simulink model "control_algorithm"  (R2021a)
settings: Solver=FixedStepDiscrete  StartTime=0.0  StopTime=Inf  FixedStep=5e-05  MaxStep=1e-6  RelTol=1e-9  EnableMultiTasking=on
values from neighbouring files (symbols this model uses):
  HW_TS = PWM_PRD    (= 5e-05)    [parameters.m]
  PWM_TIM_BASE_PRD = PWM_CPU_CLK/PWM_FS    (= 5000)    [parameters.m]
  VSI_AMP = 6    [parameters.m]
  VSI_FREQ = 50    [parameters.m]
settings Model: ExtModeTrigDuration=8  Creator=61301765  LastModifiedBy=61301765
settings SolverCC: ZeroCrossAlgorithm=Adaptive
settings DataIOCC: SaveOutput=off  SaveTime=off
settings OptimizationCC: DefaultUnderspecifiedDataType=single  EnhancedBackFolding=on  PassReuseOutputArgsAs=Individual arguments  MaxStackSize=1024  OptimizeBlockOrder=speed  DifferentSizesBufferReuse=on  OptimizationCustomize=off  DenormalBehavior=FlushToZero  EfficientTunableParamExpr=on
settings DebuggingCC: ParameterTunabilityLossMsg=error
settings HardwareCC: ProdBitPerChar=16  ProdBitPerInt=16  ProdBitPerPointer=32  ProdBitPerSizeT=32  ProdBitPerPtrDiffT=32  ProdLargestAtomicInteger=Integer  ProdLargestAtomicFloat=None  ProdWordSize=16  ProdLongLongMode=on  ProdHWDeviceType=Texas Instruments->C2000
settings SFSimCC: MATLABDynamicMemAlloc=off
settings RTWCC: SystemTargetFile=ert.tlc  HardwareBoard=TI Piccolo F280049C LaunchPad  TemplateMakefile=ert_default_tmf  Toolchain=Microsoft Visual C++ 2019 v16.0 | nmake (64-bit Windows)  PortableWordSizes=on
settings CodeAppCC: ForceParamTrailComments=on  IgnoreCustomStorageClasses=off  OperatorAnnotations=on  SimulinkDataObjDesc=on  SFDataObjDesc=on  InsertBlockDesc=on
settings ERTTargetCC: CodeReplacementLibrary=TI C28x  ExtModeTransport=3  ExtModeStaticAllocSize=5000
settings SimscapeCC: SimscapeLogType=all  SimscapeLogToSDI=on  SimscapeLogLimitData=off

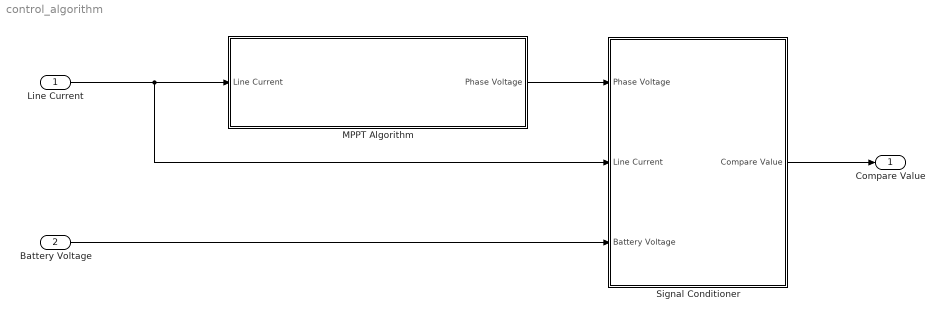
== system control_algorithm ==
  Line Current : Inport  OutDataTypeStr=double  PortDimensions=3  SampleTime=[5.0000000000000002e-05,0]
  Battery Voltage : Inport  Port=2  OutDataTypeStr=double  PortDimensions=1  SampleTime=[5.0000000000000002e-05,0]
  MPPT Algorithm : Subsystem
  Signal Conditioner : Subsystem
  Compare Value : Outport  OutDataTypeStr=uint32  PortDimensions=3  SampleTime=[5.0000000000000002e-05,0]
  wires:
  MPPT Algorithm/1(Phase Voltage) -> Signal Conditioner/1(Phase Voltage)
  Line Current/1 -> Signal Conditioner/2(Line Current), MPPT Algorithm/1(Line Current)
  Battery Voltage/1 -> Signal Conditioner/3(Battery Voltage)
  Signal Conditioner/1(Compare Value) -> Compare Value/1

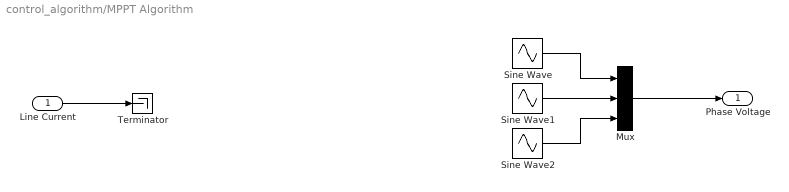
== system control_algorithm/MPPT Algorithm ==
  Line Current : Inport
  Mux : Mux  Inputs=3
  Sine Wave : Sin  Amplitude=VSI_AMP  Frequency=VSI_FREQ*2*pi  SampleTime=HW_TS  mask(DiscretizedSource){}
      mask init:
      | %zoh
  Sine Wave1 : Sin  Amplitude=VSI_AMP  Frequency=VSI_FREQ*2*pi  Phase=2*pi/3  SampleTime=HW_TS  mask(DiscretizedSource){}
      mask init:
      | %zoh
  Sine Wave2 : Sin  Amplitude=VSI_AMP  Frequency=VSI_FREQ*2*pi  Phase=-2*pi/3  SampleTime=HW_TS  mask(DiscretizedSource){}
      mask init:
      | %zoh
  Terminator : Terminator
  Phase Voltage : Outport
  wires:
  Line Current/1 -> Terminator/1
  Mux/1 -> Phase Voltage/1
  Sine Wave2/1 -> Mux/3
  Sine Wave/1 -> Mux/1
  Sine Wave1/1 -> Mux/2

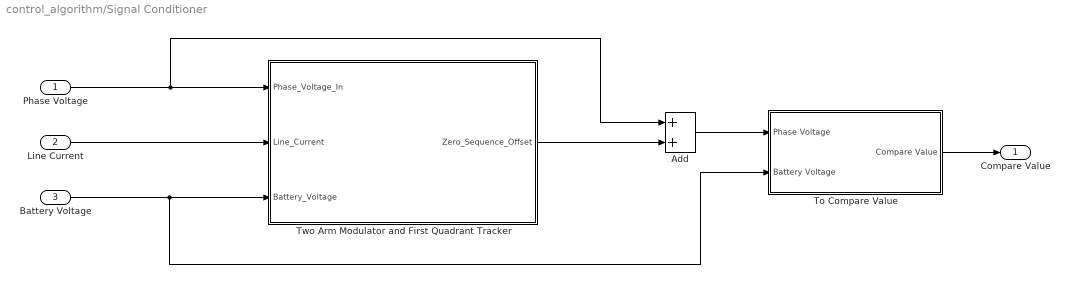
== system control_algorithm/Signal Conditioner ==
  Phase Voltage : Inport
  Line Current : Inport  Port=2
  Battery Voltage : Inport  Port=3
  Add : Sum
  To Compare Value : Subsystem
  Two Arm Modulator and First Quadrant Tracker : Stateflow chart  TreatAsAtomicUnit=on
  Compare Value : Outport
  wires:
  Phase Voltage/1 -> Two Arm Modulator and First Quadrant Tracker/1(Phase_Voltage_In), Add/1
  Battery Voltage/1 -> To Compare Value/2(Battery Voltage), Two Arm Modulator and First Quadrant Tracker/3(Battery_Voltage)
  Two Arm Modulator and First Quadrant Tracker/1(Zero_Sequence_Offset) -> Add/2
  Line Current/1 -> Two Arm Modulator and First Quadrant Tracker/2(Line_Current)
  To Compare Value/1(Compare Value) -> Compare Value/1
  Add/1 -> To Compare Value/1(Phase Voltage)

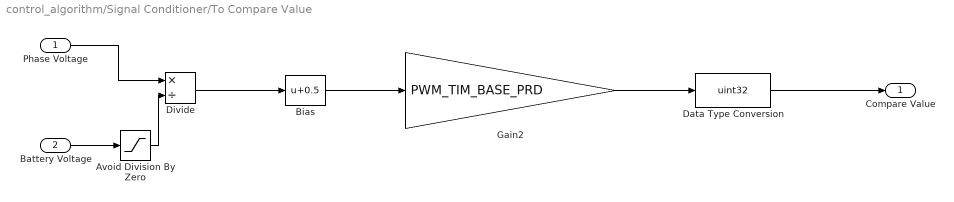
== system control_algorithm/Signal Conditioner/To Compare Value ==
  Phase Voltage : Inport
  Battery Voltage : Inport  Port=2
  Avoid Division By Zero : Saturate  UpperLimit=24  LowerLimit=0.1
  Bias : Bias  Bias=0.5
  Data Type Conversion : DataTypeConversion  OutDataTypeStr=uint32  SaturateOnIntegerOverflow=on
  Divide : Product  Inputs=*/
  Gain2 : Gain  Gain=PWM_TIM_BASE_PRD
  Compare Value : Outport
  wires:
  Data Type Conversion/1 -> Compare Value/1
  Battery Voltage/1 -> Avoid Division By Zero/1
  Divide/1 -> Bias/1
  Avoid Division By Zero/1 -> Divide/2
  Phase Voltage/1 -> Divide/1
  Gain2/1 -> Data Type Conversion/1
  Bias/1 -> Gain2/1

== stateflow chart control_algorithm/Signal Conditioner/Two Arm Modulator and First Quadrant Tracker ==
  state parallelState
    entry:
    done = false;
    state FindMaxPhase [parallel]
      settings: executionOrder=1
      (default) -> (junction 151) : % find phase at which the magnitude is maximum
      (junction 151) -> (junction 152) [order 1] : [Phase_Voltage_In(1) >= Phase_Voltage_In(2) && Phase_Voltage_In(1) >= Phase_Voltage_In(3)]
      (junction 151) -> (junction 153) [order 2]
      (junction 152) -> (junction 160) : {maxPhase = 1;}
      (junction 153) -> (junction 154) [order 1] : [Phase_Voltage_In(2) >= Phase_Voltage_In(1) && Phase_Voltage_In(2) >= Phase_Voltage_In(3)]
      (junction 153) -> (junction 155) [order 2]
      (junction 154) -> (junction 159) : {maxPhase = 2;}
      (junction 155) -> (junction 156) [order 1] : [Phase_Voltage_In(3) >= Phase_Voltage_In(1) && Phase_Voltage_In(3) >= Phase_Voltage_In(2)]
      (junction 155) -> (junction 157) [order 2] : {maxPhase = 0;}
      (junction 156) -> (junction 158) : {maxPhase = 3;}
      (junction 158) -> (junction 157)
      (junction 159) -> (junction 158)
      (junction 160) -> (junction 159)
      (junction 157) -> (junction 161)
      (junction 161) -> (junction 259) : % check whether the upper switch is operated in Q1
      (junction 259) -> (junction 257) [order 1] : [Line_Current(maxPhase) >= 0]
      (junction 259) -> (junction 260) [order 2] : {isUpperInQ1 = false;}
      (junction 257) -> (junction 261) : {isUpperInQ1 = true;}
      (junction 261) -> (junction 260)
      (junction 260) -> (junction 252)
    state FindMinPhase [parallel]
      settings: executionOrder=3
      (default) -> (junction 189) : % find phase at which the magnitude is maximum
      (junction 189) -> (junction 190) [order 1] : [Phase_Voltage_In(1) <= Phase_Voltage_In(2) && Phase_Voltage_In(1) <= Phase_Voltage_In(3)]
      (junction 189) -> (junction 191) [order 2]
      (junction 190) -> (junction 198) : {minPhase = 1;}
      (junction 191) -> (junction 192) [order 1] : [Phase_Voltage_In(2) <= Phase_Voltage_In(1) && Phase_Voltage_In(2) <= Phase_Voltage_In(3)]
      (junction 191) -> (junction 193) [order 2]
      (junction 192) -> (junction 197) : {minPhase = 2;}
      (junction 193) -> (junction 194) [order 1] : [Phase_Voltage_In(3) <= Phase_Voltage_In(1) && Phase_Voltage_In(3) <= Phase_Voltage_In(2)]
      (junction 193) -> (junction 195) [order 2] : {minPhase = 0;}
      (junction 194) -> (junction 196) : {minPhase = 3;}
      (junction 196) -> (junction 195)
      (junction 197) -> (junction 196)
      (junction 198) -> (junction 197)
      (junction 195) -> (junction 266) : % check whether the lower switch is operated in Q1
      (junction 266) -> (junction 275) [order 1] : [Line_Current(minPhase) <= 0]
      (junction 266) -> (junction 273) [order 2] : {isLowerInQ1 = false;}
      (junction 275) -> (junction 269) : {isLowerInQ1 = true;}
      (junction 269) -> (junction 273)
      (junction 273) -> (junction 267)
    state ComputeOffset [parallel]
      settings: executionOrder=2
      state TypeOne
        entry:
        Zero_Sequence_Offset = (Battery_Voltage / 2) - max(Phase_Voltage_In);
        switchCount = switchCount + 1;
      state TypeTwo
        entry:
        Zero_Sequence_Offset = - (Battery_Voltage / 2) - min(Phase_Voltage_In) ;
        switchCount = switchCount - 1;
      (default) -> (junction 227) : % decide whether to use upper or lower switch
      (junction 227) -> (junction 228) [order 1] : [isUpperInQ1 == 1 && isLowerInQ1 == 0]
      (junction 227) -> (junction 229) [order 2]
      (junction 228) -> (junction 233) : {switchCommand = 1;}
      (junction 229) -> (junction 230) [order 1] : [isUpperInQ1 == 0 && isLowerInQ1 == 1]
      (junction 229) -> (junction 231) [order 2] : {switchCommand = 3;}
      (junction 230) -> (junction 232) : {switchCommand = 2;}
      (junction 232) -> (junction 231)
      (junction 233) -> (junction 232)
      (junction 231) -> (junction 310)
      (junction 310) -> (junction 311) [order 1] : [switchCount > 5000]
      (junction 310) -> (junction 312) [order 2]
      (junction 311) -> (junction 316) : {switchCount = -1;}
      (junction 312) -> (junction 313) [order 1] : [switchCount < -5000]
      (junction 312) -> (junction 314) [order 2]
      (junction 313) -> (junction 315) : {switchCount = 1;}
      (junction 315) -> (junction 314)
      (junction 316) -> (junction 315)
      (junction 314) -> (junction 234) : {done = true;}
      (junction 234) -> (junction 282) [order 1] : [switchCommand == 2]
      (junction 234) -> (junction 283) [order 2] : [switchCommand == 1]
      (junction 234) -> (junction 289) [order 3] : % load   balancing}
      (junction 282) -> TypeTwo
      (junction 283) -> TypeOne
      (junction 289) -> (junction 283) [order 2]
      (junction 289) -> (junction 282) [order 1] : [switchCount < 0]
  (default) -> parallelState
  parallelState -> parallelState : [done]
  data: Phase_Voltage_In input; Line_Current input double size=3; Zero_Sequence_Offset output double size=1; maxPhase local int32 size=1; isLowerInQ1 local boolean size=1; isUpperInQ1 local boolean size=1; minPhase local int32 size=1; switchCommand local int32 size=1 =int32(0); done local boolean; Battery_Voltage input; switchCount local =0
